simulink model "IMU_Reader_R2018b"  (R2018b)
settings: Solver=VariableStepAuto  StartTime=0.0  StopTime=inf  RelTol=1e-3
InitFcn:
  | Ts=0.1;
libraries: instrumentlib x2
settings Model: Creator=amind  LastModifiedBy=amind
settings DataIOCC: ReturnWorkspaceOutputs=on
settings ConfigComp: CovBoundaryAbsTol=1.0e-5

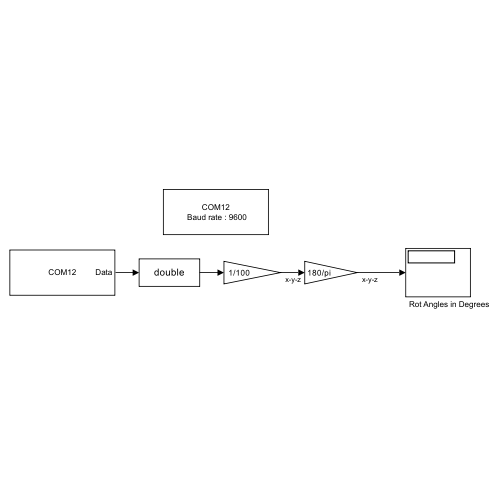
[thumbnail: Simulink's stored preview of the top-level diagram]
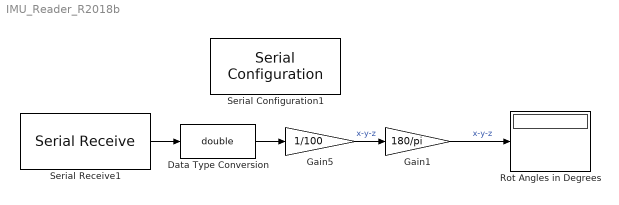
== system IMU_Reader_R2018b ==
  "          Rot Angles in Degrees" : Display
  Data Type Conversion : DataTypeConversion  OutDataTypeStr=double
  Gain1 : Gain  Gain=180/pi
  Gain5 : Gain  Gain=1/100
  Serial Configuration1 : instrumentlib/Serial Configuration  Priority=-200000  ObjConstructor="\"serial('COM12');\""  ComPortMenu=COM12  ComPort=COM12  BaudRate=9600  DataBits=8  Parity=none  StopBits=1  ByteOrder=LittleEndian  FlowControl=none  Timeout=60
  Serial Receive1 : instrumentlib/Serial Receive  Priority=1  ObjConstructor="\"serial('COM12');\""  ComPortMenu=COM12  ComPort=COM12  DataType=int16  DataSize=[3 1]  EnableBlockingMode=on  ActionDataUnavailable=Output last received value  CustomValue=0  SampleTime=Ts
  wires:
  Serial Receive1/1 -> Data Type Conversion/1
  Data Type Conversion/1 -> Gain5/1
  Gain5/1 -> Gain1/1  "x-y-z"
  Gain1/1 -> "          Rot Angles in Degrees"/1  "x-y-z"
